simulink model "BMS_Harness_PowerCalc"  (R2025b)
settings: configuration reference "AutosarConfig" (kept outside this file)
undefined symbols (not defined in the file or in its folder): SRE
libraries: SignalEditorBlockLib x1
settings Model: DataDictionary=BMS_Software_DD.sldd  Creator=smuckati  LastModifiedBy=smuckati
settings ConfigSetRef: SourceName=AutosarConfig

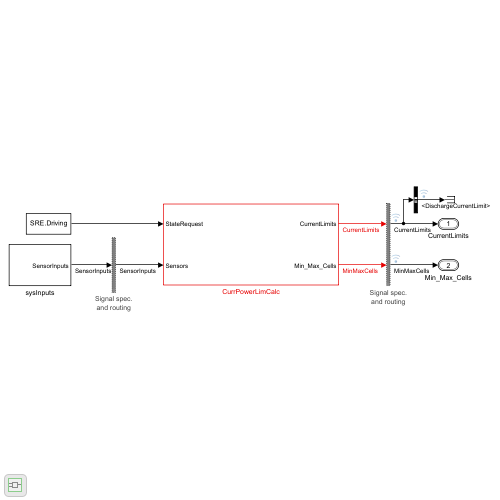
[thumbnail: Simulink's stored preview of the top-level diagram]
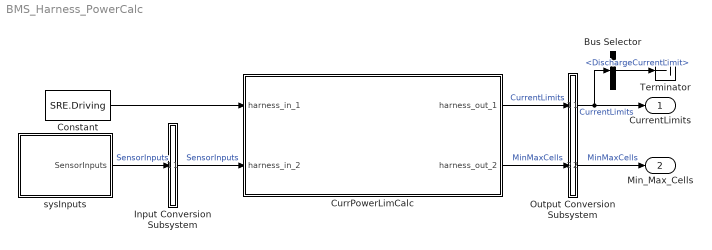
== system BMS_Harness_PowerCalc ==
  Bus Selector : BusSelector  OutputSignals=DischargeCurrentLimit
  Constant : Constant  Value=SRE.Driving
  CurrPowerLimCalc : Subsystem  Tag=__SL_testing_harness_stub_
  Input Conversion Subsystem : Subsystem  Tag=__SLT_ICS__  Description=|
      | Signal spec.
      | and routing
      settings: AttributesFormatString=%<Description>
  Output Conversion Subsystem : Subsystem  Tag=__SLT_OCS__  Description=|
      | Signal spec.
      | and routing
      settings: AttributesFormatString=%<Description>
  Terminator : Terminator
  sysInputs : Subsystem
  CurrentLimits : Outport  OutDataTypeStr=Bus: CurrentLimits
  Min_Max_Cells : Outport  Port=2  OutDataTypeStr=Bus: Min_Max_Cells
  wires:
  Output Conversion Subsystem/1(Outport_1) -> Bus Selector/1, CurrentLimits/1  "CurrentLimits"
  Output Conversion Subsystem/2(Outport_2) -> Min_Max_Cells/1  "MinMaxCells"
  Input Conversion Subsystem/1(Outport_1) -> CurrPowerLimCalc/2(harness_in_2)  "SensorInputs"
  CurrPowerLimCalc/1(harness_out_1) -> Output Conversion Subsystem/1(Inport_1)  "CurrentLimits"
  CurrPowerLimCalc/2(harness_out_2) -> Output Conversion Subsystem/2(Inport_2)  "MinMaxCells"
  sysInputs/1(SensorInputs) -> Input Conversion Subsystem/1(Inport_1)  "SensorInputs"
  Bus Selector/1 -> Terminator/1  "<DischargeCurrentLimit>"
  Constant/1 -> CurrPowerLimCalc/1(harness_in_1)

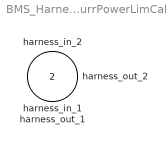
== system BMS_Harness_PowerCalc/CurrPowerLimCalc ==
  harness_in_1 : Inport
  harness_in_2 : Inport  Port=2
  harness_out_1 : Outport
  harness_out_2 : Outport  Port=2

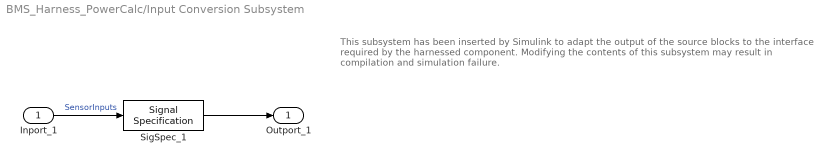
== system BMS_Harness_PowerCalc/Input Conversion Subsystem ==
  note: This subsystem has been inserted by Simulink to adapt the output of the source blocks to the interface required by the harnessed component.
      |  Modifying the contents of this subsystem may result in compilation and simulation failure.
  Inport_1 : Inport
  SigSpec_1 : SignalSpecification  OutDataTypeStr=Bus: Sensors  Dimensions=[1]  SampleTime=0.1  BusOutputAsStruct=on
  Outport_1 : Outport
  wires:
  SigSpec_1/1 -> Outport_1/1
  Inport_1/1 -> SigSpec_1/1  "SensorInputs"

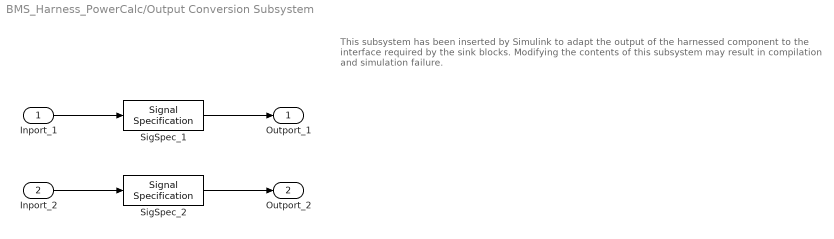
== system BMS_Harness_PowerCalc/Output Conversion Subsystem ==
  note: This subsystem has been inserted by Simulink to adapt the output of the harnessed component to the interface required by the sink blocks.
      |  Modifying the contents of this subsystem may result in compilation and simulation failure.
  Inport_1 : Inport
  Inport_2 : Inport  Port=2
  SigSpec_1 : SignalSpecification  OutDataTypeStr=Bus: CurrentLimits  Dimensions=[1]  SampleTime=0.1  BusOutputAsStruct=on
  SigSpec_2 : SignalSpecification  OutDataTypeStr=Bus: Min_Max_Cells  Dimensions=[1]  SampleTime=0.1  BusOutputAsStruct=on
  Outport_1 : Outport
  Outport_2 : Outport  Port=2
  wires:
  Inport_1/1 -> SigSpec_1/1
  SigSpec_1/1 -> Outport_1/1
  Inport_2/1 -> SigSpec_2/1
  SigSpec_2/1 -> Outport_2/1

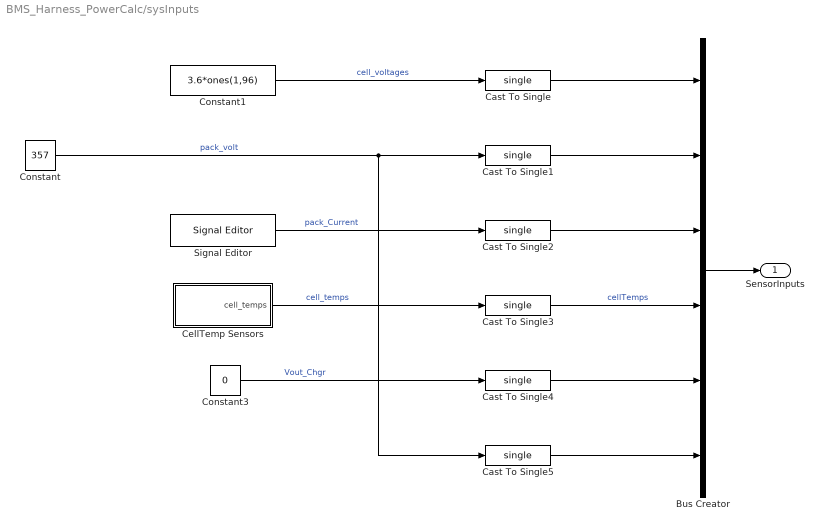
== system BMS_Harness_PowerCalc/sysInputs ==
  Bus Creator : BusCreator  Inputs=6  OutDataTypeStr=Bus: Sensors  NonVirtualBus=on
      settings: InheritFromInputs=off
  Cast To Single{,1..5} (6 alike) : DataTypeConversion  OutDataTypeStr=single  SaturateOnIntegerOverflow=off  RndMeth=Floor
  CellTemp Sensors : Subsystem
  Constant : Constant  Value=357
  Constant1 : Constant  Value=3.6*ones(1,96)
  Constant3 : Constant  Value=0
  Signal Editor : SignalEditorBlockLib/Signal Editor  FileName=PowerCalc_HarnessInputs.mat  ActiveScenario=Scenario  ActiveSignal=PackCurrent  IsBus=off  OutputBusObjectStr=Bus: BusObject  SampleTime=0  Interpolate=off  ZeroCross=off  OutputAfterFinalValue=Setting to zero  Unit=inherit  PreserveSignalName=on  ApplySigPropsToAllScenarios=on  ApplySigPropsToAllSignals=off  SignalPropertySource=Dialog parameters
  SensorInputs : Outport
  wires:
  Bus Creator/1 -> SensorInputs/1
  Constant1/1 -> Cast To Single/1  "cell_voltages"
  Constant/1 -> Cast To Single5/1, Cast To Single1/1  "pack_volt"
  Constant3/1 -> Cast To Single4/1  "Vout_Chgr"
  Signal Editor/1 -> Cast To Single2/1  "pack_Current"
  Cast To Single/1 -> Bus Creator/1
  Cast To Single1/1 -> Bus Creator/2
  Cast To Single2/1 -> Bus Creator/3
  Cast To Single3/1 -> Bus Creator/4  "cellTemps"
  Cast To Single4/1 -> Bus Creator/5
  Cast To Single5/1 -> Bus Creator/6
  CellTemp Sensors/1(cell_temps) -> Cast To Single3/1  "cell_temps"

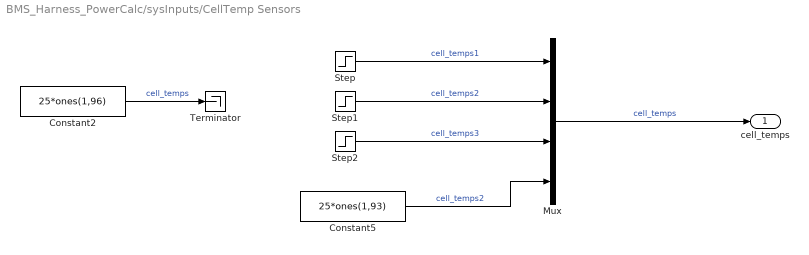
== system BMS_Harness_PowerCalc/sysInputs/CellTemp Sensors ==
  Constant2 : Constant  Value=25*ones(1,96)
  Constant5 : Constant  Value=25*ones(1,93)
  Mux : Mux
  Step : Step  Time=400  Before=24  After=14  SampleTime=0
      settings: AttributesFormatString=Tfinal = 14
  Step1 : Step  Time=400  Before=24  After=14  SampleTime=0
      settings: AttributesFormatString=Tfinal = 14
  Step2 : Step  Time=400  Before=24  After=12  SampleTime=0
      settings: AttributesFormatString=Tfinal = 12
  Terminator : Terminator
  cell_temps : Outport
  wires:
  Constant5/1 -> Mux/4  "cell_temps2"
  Constant2/1 -> Terminator/1  "cell_temps"
  Step1/1 -> Mux/2  "cell_temps2"
  Mux/1 -> cell_temps/1  "cell_temps"
  Step/1 -> Mux/1  "cell_temps1"
  Step2/1 -> Mux/3  "cell_temps3"
